simulink model "Test_Byte_Multiplexer_8_to_1"  (Simulink 8.1)
settings: Solver=ode45  StartTime=0.0  StopTime=len  RelTol=1e-3
libraries: Byte_Multiplexers_Lib x1, commutil2 x1
settings Model: Creator=N  LastModifiedBy=uzivatel
settings DataIOCC: LimitDataPoints=off  SignalLoggingSaveFormat=Dataset
settings OptimizationCC: ExpressionDepthLimit=128
settings DebuggingCC: UnderspecifiedInitializationDetection=Simplified  MergeDetectMultiDrivingBlocksExec=error  SolverPrmCheckMsg=none  FcnCallInpInsideContextMsg=EnableAllAsError  FrameProcessingCompatibilityMsg=error  StateNameClashWarn=none
settings HardwareCC: ProdBitPerPointer=64  ProdLargestAtomicFloat=Float  ProdIntDivRoundTo=Zero  ProdEndianess=LittleEndian  ProdHWDeviceType=Intel->x86-64 (Windows64)
settings ModelReferenceCC: PropagateSignalLabelsOutOfModel=on
settings GRTTargetCC: CodeReplacementLibrary=None  CombineOutputUpdateFcns=on  CPPClassGenCompliant=on  GRTInterface=off

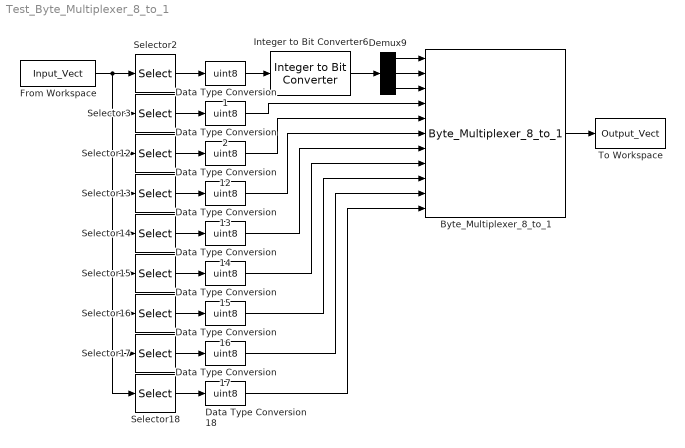
== system Test_Byte_Multiplexer_8_to_1 ==
  Byte_Multiplexer_8_to_1 : Byte_Multiplexers_Lib/Byte_Multiplexers_Lib/Byte_Multiplexer_8_to_1
  Data Type Conversion{1..2,12..18} (9 alike) : DataTypeConversion  OutDataTypeStr=uint8
  Demux9 : Demux  Outputs=3
  From Workspace : FromWorkspace  VariableName=Input_Vect  SampleTime=1  Interpolate=off  OutputAfterFinalValue=Holding final value
  Integer to Bit Converter6 : commutil2/Integer to Bit Converter  nbits=3  signedInputValues=Unsigned  bitOrder=MSB first  outDtype=boolean
  Selector12 : Selector  IndexMode=Zero-based  InputPortWidth=9  IndexOptions=Index vector (dialog)  Indices=2  OutputSizes=1
  Selector13 : Selector  IndexMode=Zero-based  InputPortWidth=9  IndexOptions=Index vector (dialog)  Indices=3  OutputSizes=1
  Selector14 : Selector  IndexMode=Zero-based  InputPortWidth=9  IndexOptions=Index vector (dialog)  Indices=4  OutputSizes=1
  Selector15 : Selector  IndexMode=Zero-based  InputPortWidth=9  IndexOptions=Index vector (dialog)  Indices=5  OutputSizes=1
  Selector16 : Selector  IndexMode=Zero-based  InputPortWidth=9  IndexOptions=Index vector (dialog)  Indices=6  OutputSizes=1
  Selector17 : Selector  IndexMode=Zero-based  InputPortWidth=9  IndexOptions=Index vector (dialog)  Indices=7  OutputSizes=1
  Selector18 : Selector  IndexMode=Zero-based  InputPortWidth=9  IndexOptions=Index vector (dialog)  Indices=8  OutputSizes=1
  Selector2 : Selector  IndexMode=Zero-based  InputPortWidth=9  SampleTime=1  IndexOptions=Index vector (dialog)  Indices=0  OutputSizes=1
  Selector3 : Selector  IndexMode=Zero-based  InputPortWidth=9  IndexOptions=Index vector (dialog)  Indices=1  OutputSizes=1
  To Workspace : ToWorkspace  VariableName=Output_Vect  SampleTime=1
  wires:
  Byte_Multiplexer_8_to_1/1 -> To Workspace/1
  Demux9/1 -> Byte_Multiplexer_8_to_1/1
  Demux9/2 -> Byte_Multiplexer_8_to_1/2
  Demux9/3 -> Byte_Multiplexer_8_to_1/3
  Integer to Bit Converter6/1 -> Demux9/1
  From Workspace/1 -> Selector12/1, Selector13/1, Selector14/1, Selector15/1, Selector16/1, Selector17/1, Selector18/1, Selector3/1, Selector2/1
  Selector2/1 -> Data Type Conversion1/1
  Selector3/1 -> Data Type Conversion2/1
  Data Type Conversion1/1 -> Integer to Bit Converter6/1
  Data Type Conversion2/1 -> Byte_Multiplexer_8_to_1/4
  Selector12/1 -> Data Type Conversion12/1
  Selector13/1 -> Data Type Conversion13/1
  Selector14/1 -> Data Type Conversion14/1
  Selector15/1 -> Data Type Conversion15/1
  Selector16/1 -> Data Type Conversion16/1
  Selector17/1 -> Data Type Conversion17/1
  Selector18/1 -> Data Type Conversion18/1
  Data Type Conversion12/1 -> Byte_Multiplexer_8_to_1/5
  Data Type Conversion13/1 -> Byte_Multiplexer_8_to_1/6
  Data Type Conversion14/1 -> Byte_Multiplexer_8_to_1/7
  Data Type Conversion15/1 -> Byte_Multiplexer_8_to_1/8
  Data Type Conversion16/1 -> Byte_Multiplexer_8_to_1/9
  Data Type Conversion17/1 -> Byte_Multiplexer_8_to_1/10
  Data Type Conversion18/1 -> Byte_Multiplexer_8_to_1/11
